simulink library "QuatSixDoFDynamics_ul"  (R2018b)
settings: Solver=VariableStepAuto  StartTime=0.0  StopTime=10.0  RelTol=1e-3
undefined symbols (not defined in the file): initAngRates, Jinv, Jtot, Minv
libraries: sharedtransform x3, vrlib x2
settings Model: Creator=mcobb  LastModifiedBy=asiddiq2

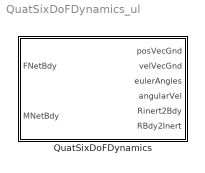
== system QuatSixDoFDynamics_ul ==
  QuatSixDoFDynamics : Subsystem  mask{M=1, M_added=zeros(3,3), J=eye(3), J_added=zeros(3,3), initPos=0, initVel=0, initEulAngs=0, initAngVel=0}
      mask prompts: M "Mass"; M_added "Added mass matrix"; J "Inertia matrix"; J_added "Added inertia matrix"; initPos "Initial position"; initVel "Initial velocity"; initEulAngs "Initial Euler Angles"; initAngVel "Initial Angular Velocity Vec"
      mask init:
      | sixDoFDynamics_init

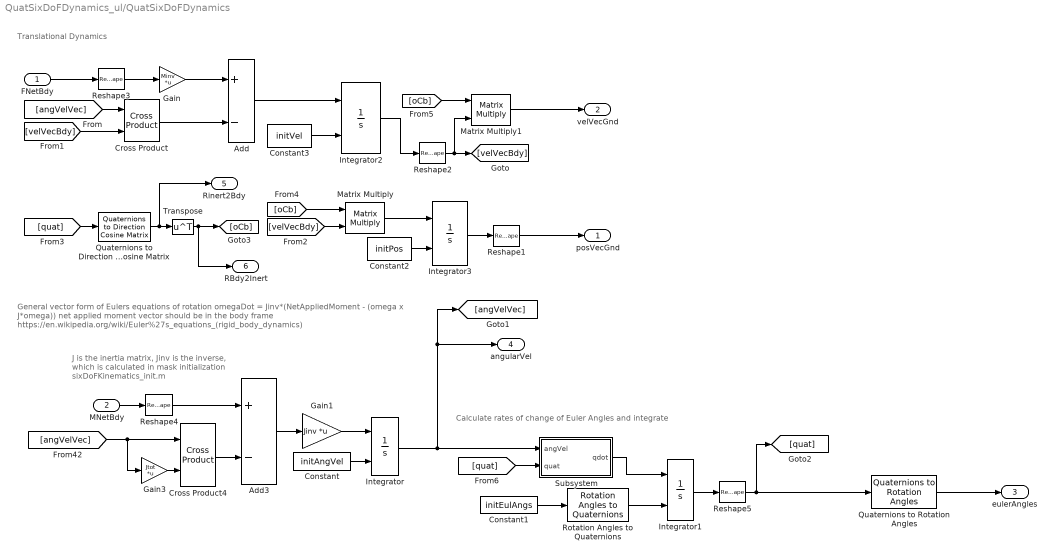
== system QuatSixDoFDynamics_ul/QuatSixDoFDynamics ==
  note: Translational Dynamics
  note: Calculate rates of change of Euler Angles and integrate
  note: General vector form of Eulers equations of rotation
      | omegaDot = Jinv*(NetAppliedMoment - (omega x J*omega))
      | net applied moment vector should be in the body frame
      | https://en.wikipedia.org/wiki/Euler%27s_equations_(rigid_body_dynamics)
  note: J is the inertia matrix, Jinv is the inverse,
      | which is calculated in mask initialization
      | sixDoFKinematics_init.m
  FNetBdy : Inport
  MNetBdy : Inport  Port=2
  Add : Sum  Inputs=+-
  Add3 : Sum  Inputs=+-
  Constant : Constant  Value=initAngVel
  Constant1 : Constant  Value=initEulAngs
  Constant2 : Constant  Value=initPos
  Constant3 : Constant  Value=initVel
  Cross Product : vrlib/Utilities/Cross Product
      settings: SourceProductBaseCode=VR
  Cross Product4 : vrlib/Utilities/Cross Product
      settings: SourceProductBaseCode=VR
  Gain : Gain  Gain=Minv  Multiplication=Matrix(K*u)
  Gain1 : Gain  Gain=Jinv  Multiplication=Matrix(K*u)
  Gain3 : Gain  Gain=Jtot  Multiplication=Matrix(K*u)
  Integrator : Integrator  InitialConditionSource=external  InitialCondition=initAngRates
  Integrator1 : Integrator  InitialConditionSource=external  InitialCondition=initEulAngs
  Integrator2 : Integrator  InitialConditionSource=external  InitialCondition=initVel
  Integrator3 : Integrator  InitialConditionSource=external  InitialCondition=initPos
  Matrix Multiply : Product  Multiplication=Matrix(*)
  Matrix Multiply1 : Product  Multiplication=Matrix(*)
  Quaternions to Direction Cosine Matrix : sharedtransform/Quaternions to  Direction Cosine Matrix  aMode=aMode
      settings: SourceProductName=Aerospace Blockset  SourceProductBaseCode=AE
  Quaternions to Rotation Angles : sharedtransform/Quaternions to Rotation Angles  rotationOrder=XYZ  aMode=aMode
      settings: SourceProductBaseCode=AE
  Reshape{1..5} (5 alike) : Reshape  OutputDimensionality=Column vector (2-D)
  Rotation Angles to Quaternions : sharedtransform/Rotation Angles to Quaternions  rotationOrder=XYZ  aMode=aMode
      settings: SourceProductName=Aerospace Blockset  SourceProductBaseCode=AE
  Subsystem : Subsystem
  Transpose : Math  Operator=transpose  SaturateOnIntegerOverflow=on
  posVecGnd : Outport
  velVecGnd : Outport  Port=2
  eulerAngles : Outport  Port=3
  angularVel : Outport  Port=4
  Rinert2Bdy : Outport  Port=5
  RBdy2Inert : Outport  Port=6
  wires:
  Reshape4/1 -> Add3/1
  Gain/1 -> Add/1
  [oCb] -> Matrix Multiply1/1
  Reshape1/1 -> posVecGnd/1
  Constant3/1 -> Integrator2/2
  Matrix Multiply1/1 -> velVecGnd/1
  [oCb] -> Matrix Multiply/1
  Cross Product4/1 -> Add3/2
  Integrator1/1 -> Reshape5/1
  Integrator/1 -> Subsystem/1(angVel), angularVel/1, [angVelVec]
  MNetBdy/1 -> Reshape4/1
  Cross Product/1 -> Add/2
  Add/1 -> Integrator2/1
  [velVecBdy] -> Cross Product/2
  Matrix Multiply/1 -> Integrator3/1
  Add3/1 -> Gain1/1
  Reshape3/1 -> Gain/1
  [velVecBdy] -> Matrix Multiply/2
  Reshape5/1 -> Quaternions to Rotation Angles/1, [quat]
  [angVelVec] -> Cross Product4/1, Gain3/1
  Constant2/1 -> Integrator3/2
  Integrator2/1 -> Reshape2/1
  FNetBdy/1 -> Reshape3/1
  Subsystem/1(qdot) -> Integrator1/1
  [angVelVec] -> Cross Product/1
  Gain3/1 -> Cross Product4/2
  Reshape2/1 -> Matrix Multiply1/2, [velVecBdy]
  Constant/1 -> Integrator/2
  Constant1/1 -> Rotation Angles to Quaternions/1
  Gain1/1 -> Integrator/1
  Integrator3/1 -> Reshape1/1
  [quat] -> Quaternions to Direction Cosine Matrix/1
  Rotation Angles to Quaternions/1 -> Integrator1/2
  Quaternions to Rotation Angles/1 -> eulerAngles/1
  [quat] -> Subsystem/2(quat)
  Transpose/1 -> RBdy2Inert/1, [oCb]
  Quaternions to Direction Cosine Matrix/1 -> Rinert2Bdy/1, Transpose/1

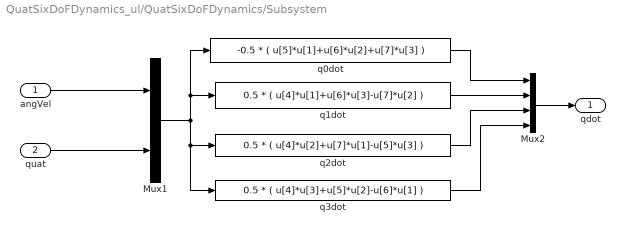
== system QuatSixDoFDynamics_ul/QuatSixDoFDynamics/Subsystem ==
  angVel : Inport
  quat : Inport  Port=2
  Mux1 : Mux  Inputs=[3 4]
  Mux2 : Mux
  q0dot : Fcn  Expr=-0.5 * ( u[5]*u[1]+u[6]*u[2]+u[7]*u[3] )
  q1dot : Fcn  Expr=0.5 * ( u[4]*u[1]+u[6]*u[3]-u[7]*u[2] )
  q2dot : Fcn  Expr=0.5 * ( u[4]*u[2]+u[7]*u[1]-u[5]*u[3] )
  q3dot : Fcn  Expr=0.5 * ( u[4]*u[3]+u[5]*u[2]-u[6]*u[1] )
  qdot : Outport
  wires:
  quat/1 -> Mux1/2
  q3dot/1 -> Mux2/4
  Mux2/1 -> qdot/1
  q2dot/1 -> Mux2/3
  q1dot/1 -> Mux2/2
  q0dot/1 -> Mux2/1
  angVel/1 -> Mux1/1
  Mux1/1 -> q2dot/1, q3dot/1, q0dot/1, q1dot/1
